simulink model "Que6"  (R2023b)
settings: Solver=VariableStepAuto  StartTime=0.0  StopTime=20  FixedStep=0.0001  RelTol=1e-3
libraries: simulink x1
settings Model: Creator=ali14  LastModifiedBy=setak
settings OptimizationCC: ReuseModelBlockBuffer=off

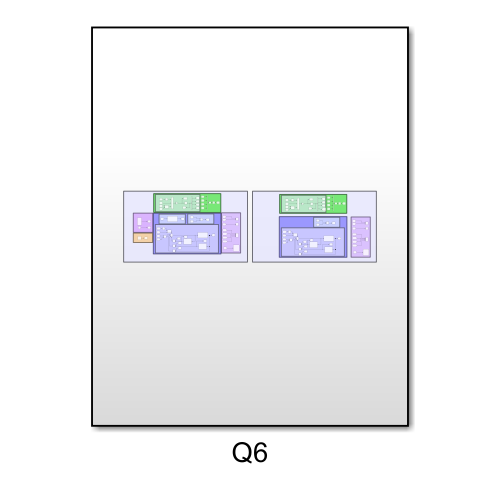
[thumbnail: Simulink's stored preview of the top-level diagram]
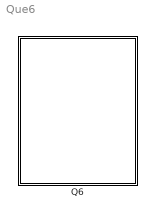
== system Que6 ==
  Q6 : Subsystem

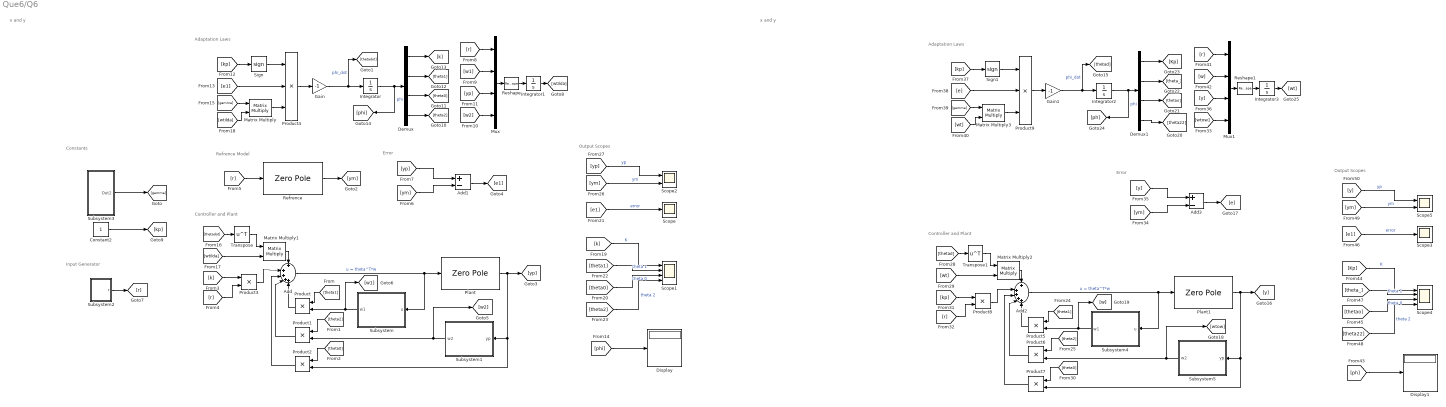
== system Que6/Q6 ==
  note: x and y
  note: Constants
  note: Input Generator
  note: Adaptation Laws
  note: Controller and Plant
  note: Error
  note: Refrence Model
  note: Output Scopes
  note: x and y
  note: Error
  note: Controller and Plant
  note: Adaptation Laws
  note: Output Scopes
  Add : Sum  Inputs=+|++++
  Add1 : Sum  Inputs=+-
  Add2 : Sum  Inputs=+|++++
  Add3 : Sum  Inputs=+-
  Constant2 : Constant
  Demux : Demux
  Demux1 : Demux
  Display : Display
  Display1 : Display
  Gain : Gain  Gain=-1
  Gain1 : Gain  Gain=-1
  Integrator{,1..3} (4 alike) : Integrator
  Matrix Multiply{,1..3} (4 alike) : Product  Multiplication=Matrix(*)
  Mux : Mux
  Mux1 : Mux
  Plant : ZeroPole  Zeros=[]  Poles=[0 0]  Gain=1/2.5
  Plant1 : ZeroPole  Zeros=[]  Poles=[0 0]  Gain=1/0.03
  Product{,1..3,5..8} (8 alike) : Product
  Product4 : Product  Inputs=3
  Product9 : Product  Inputs=3
  Refrence : ZeroPole  Zeros=[]  Poles=[-1 -1]  Gain=1
  Reshape : Reshape  OutputDimensionality=Column vector (2-D)
  Reshape1 : Reshape  OutputDimensionality=Column vector (2-D)
  Scope : Scope
  Scope1 : Scope  NumInputPorts=4
  Scope2 : Scope  NumInputPorts=2
  Scope3 : Scope
  Scope4 : Scope  NumInputPorts=4
  Scope5 : Scope  NumInputPorts=2
  Sign : Signum
  Sign1 : Signum
  Subsystem : Subsystem
  Subsystem1 : Subsystem
  Subsystem2 : Subsystem
  Subsystem3 : Subsystem
  Subsystem4 : Subsystem
  Subsystem5 : Subsystem
  Transpose : Math  Operator=transpose
  Transpose1 : Math  Operator=transpose
  wires:
  Demux/1 -> [k]
  Subsystem1/1(w2) -> Product1/2, [w2]
  [theta2] -> Product1/1
  Demux/4 -> [theta2]
  Plant/1 -> [yp], Product2/2, Subsystem1/1(yp)
  Constant2/1 -> [kp]
  Refrence/1 -> [ym]
  [kp] -> Sign/1
  [r] -> Refrence/1
  [w1] -> Mux/2
  Sign/1 -> Product4/1
  [k] -> Product3/1
  Add1/1 -> [e1]
  [yp] -> Add1/1
  [theta1] -> Product/1
  Subsystem/1(w1) -> [w1], Product/2
  Add/1 -> Subsystem/1(u), Plant/1  "u = theta^T*w"
  Mux/1 -> Reshape/1
  [w2] -> Mux/4
  Demux/3 -> [theta0]
  [r] -> Product3/2
  [ym] -> Add1/2
  [theta0] -> Product2/1
  Gain/1 -> [thetadot], Integrator/1  "phi_dot"
  Product4/1 -> Gain/1
  [r] -> Mux/1
  Integrator/1 -> [phi], Demux/1  "phi"
  Demux/2 -> [theta1]
  Subsystem2/1(r) -> [r]
  [e1] -> Product4/2
  [yp] -> Mux/3
  [wtilda] -> Matrix Multiply/2
  Matrix Multiply/1 -> Product4/3
  [gamma] -> Matrix Multiply/1
  [yp] -> Scope2/1  "yp"
  [theta1] -> Scope1/2  "theta 1"
  [theta0] -> Scope1/3  "theta 0"
  [theta2] -> Scope1/4  "theta 2"
  [e1] -> Scope/1  "error"
  [ym] -> Scope2/2  "ym"
  [k] -> Scope1/1  "K"
  Reshape/1 -> Integrator1/1
  Integrator1/1 -> [wtilda]
  Transpose/1 -> Matrix Multiply1/1
  [wtilda] -> Matrix Multiply1/2
  [thetadot] -> Transpose/1
  Product/1 -> Add/5
  Product1/1 -> Add/4
  Product2/1 -> Add/3
  Product3/1 -> Add/2
  Matrix Multiply1/1 -> Add/1
  [phi] -> Display/1
  Subsystem3/1(Out2) -> [gamma]
  Subsystem4/1(w1) -> [w], Product5/2
  Product8/1 -> Add2/2
  Product7/1 -> Add2/3
  [thetad] -> Transpose1/1
  [theta0] -> Product7/1
  Product5/1 -> Add2/5
  [y] -> Add3/1
  [ym] -> Add3/2
  [r] -> Product8/2
  Transpose1/1 -> Matrix Multiply2/1
  Add2/1 -> Subsystem4/1(u), Plant1/1  "u = theta^T*w"
  Matrix Multiply2/1 -> Add2/1
  [theta2] -> Product6/1
  [wt] -> Matrix Multiply2/2
  Product6/1 -> Add2/4
  Subsystem5/1(w2) -> Product6/2, [wtow]
  Add3/1 -> [e]
  Plant1/1 -> [y], Product7/2, Subsystem5/1(yp)
  [theta1] -> Product5/1
  [kp] -> Product8/1
  [gamma] -> Matrix Multiply3/1
  Reshape1/1 -> Integrator3/1
  Matrix Multiply3/1 -> Product9/3
  Mux1/1 -> Reshape1/1
  Demux1/4 -> [theta22]
  [y] -> Mux1/3
  Demux1/3 -> [thetao]
  [e] -> Product9/2
  Demux1/2 -> [theta_]
  Integrator2/1 -> [ph], Demux1/1  "phi"
  Integrator3/1 -> [wt]
  [wt] -> Matrix Multiply3/2
  Gain1/1 -> [thetad], Integrator2/1  "phi_dot"
  Product9/1 -> Gain1/1
  [kp] -> Sign1/1
  [r] -> Mux1/1
  Demux1/1 -> [Kp]
  [wtow] -> Mux1/4
  [w] -> Mux1/2
  Sign1/1 -> Product9/1
  [thetao] -> Scope4/3  "theta 0"
  [y] -> Scope5/1  "yp"
  [Kp] -> Scope4/1  "K"
  [ph] -> Display1/1
  [theta_] -> Scope4/2  "theta 1"
  [theta22] -> Scope4/4  "theta 2"
  [ym] -> Scope5/2  "ym"
  [e1] -> Scope3/1  "error"

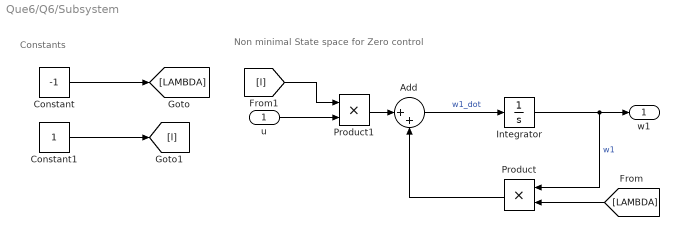
== system Que6/Q6/Subsystem ==
  note: Non minimal State space for Zero control
  note: Constants
  u : Inport
  Add : Sum  Inputs=|++
  Constant : Constant  Value=-1
  Constant1 : Constant
  Integrator : Integrator
  Product : Product
  Product1 : Product
  w1 : Outport
  wires:
  Integrator/1 -> Product/1, w1/1  "w1"
  Add/1 -> Integrator/1  "w1_dot"
  [LAMBDA] -> Product/2
  Product/1 -> Add/2
  [l] -> Product1/1
  Product1/1 -> Add/1
  u/1 -> Product1/2
  Constant1/1 -> [l]
  Constant/1 -> [LAMBDA]

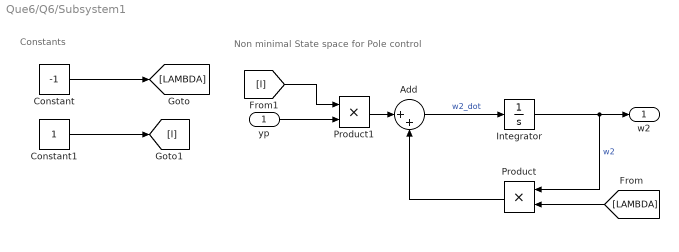
== system Que6/Q6/Subsystem1 ==
  note: Constants
  note: Non minimal State space for Pole control
  yp : Inport
  Add : Sum  Inputs=|++
  Constant : Constant  Value=-1
  Constant1 : Constant
  Integrator : Integrator
  Product : Product
  Product1 : Product
  w2 : Outport
  wires:
  Constant1/1 -> [l]
  Constant/1 -> [LAMBDA]
  [LAMBDA] -> Product/2
  [l] -> Product1/1
  Product1/1 -> Add/1
  Integrator/1 -> Product/1, w2/1  "w2"
  yp/1 -> Product1/2
  Add/1 -> Integrator/1  "w2_dot"
  Product/1 -> Add/2

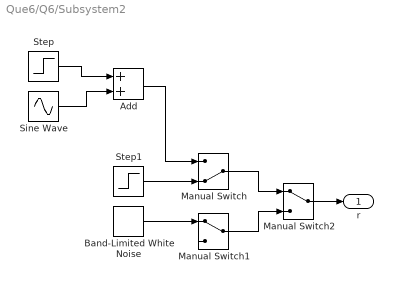
== system Que6/Q6/Subsystem2 ==
  Add : Sum
  Band-Limited White Noise : simulink/Sources/Band-Limited White Noise  Cov=[0.1]  Ts=0.1  seed=[23341]
  Manual Switch : ManualSwitch  CurrentSetting=0
  Manual Switch1 : ManualSwitch
  Manual Switch2 : ManualSwitch
  Sine Wave : Sin  SampleTime=0
  Step : Step  Time=0  SampleTime=0
  Step1 : Step  SampleTime=0
  r : Outport
  wires:
  Add/1 -> Manual Switch/1
  Step/1 -> Add/1
  Sine Wave/1 -> Add/2
  Step1/1 -> Manual Switch/2
  Manual Switch2/1 -> r/1
  Manual Switch/1 -> Manual Switch2/1
  Manual Switch1/1 -> Manual Switch2/2
  Band-Limited White Noise/1 -> Manual Switch1/1

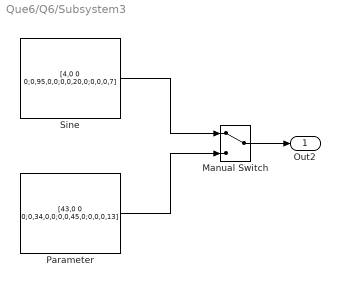
== system Que6/Q6/Subsystem3 ==
  Manual Switch : ManualSwitch
  Parameter : Constant  Value=[43,0 0 0;0,34,0,0;0,0,45,0;0,0,0,13]
  Sine : Constant  Value=[4,0 0 0;0,95,0,0;0,0,20,0;0,0,0,7]
  Out2 : Outport
  wires:
  Parameter/1 -> Manual Switch/2
  Manual Switch/1 -> Out2/1
  Sine/1 -> Manual Switch/1

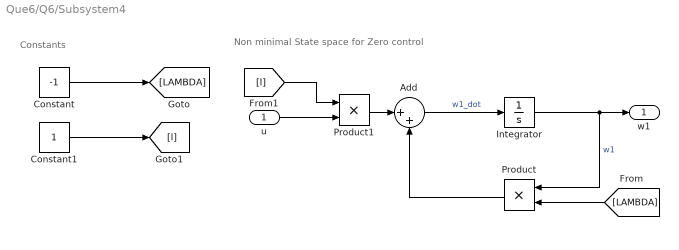
== system Que6/Q6/Subsystem4 ==
  note: Non minimal State space for Zero control
  note: Constants
  u : Inport
  Add : Sum  Inputs=|++
  Constant : Constant  Value=-1
  Constant1 : Constant
  Integrator : Integrator
  Product : Product
  Product1 : Product
  w1 : Outport
  wires:
  Integrator/1 -> Product/1, w1/1  "w1"
  Add/1 -> Integrator/1  "w1_dot"
  [LAMBDA] -> Product/2
  Product/1 -> Add/2
  [l] -> Product1/1
  Product1/1 -> Add/1
  u/1 -> Product1/2
  Constant1/1 -> [l]
  Constant/1 -> [LAMBDA]

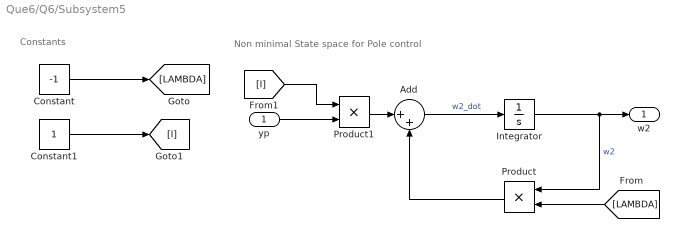
== system Que6/Q6/Subsystem5 ==
  note: Constants
  note: Non minimal State space for Pole control
  yp : Inport
  Add : Sum  Inputs=|++
  Constant : Constant  Value=-1
  Constant1 : Constant
  Integrator : Integrator
  Product : Product
  Product1 : Product
  w2 : Outport
  wires:
  Constant1/1 -> [l]
  Constant/1 -> [LAMBDA]
  [LAMBDA] -> Product/2
  [l] -> Product1/1
  Product1/1 -> Add/1
  Integrator/1 -> Product/1, w2/1  "w2"
  yp/1 -> Product1/2
  Add/1 -> Integrator/1  "w2_dot"
  Product/1 -> Add/2
